simulink library "coeffs"  (R2014a)
settings: Solver=ode45  StartTime=0.0  StopTime=10.0  RelTol=1e-3
undefined symbols (not defined in the file or in its folder): par
settings Model: Creator=goghino  LastModifiedBy=goghino

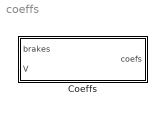
== system coeffs ==
  Coeffs : Subsystem

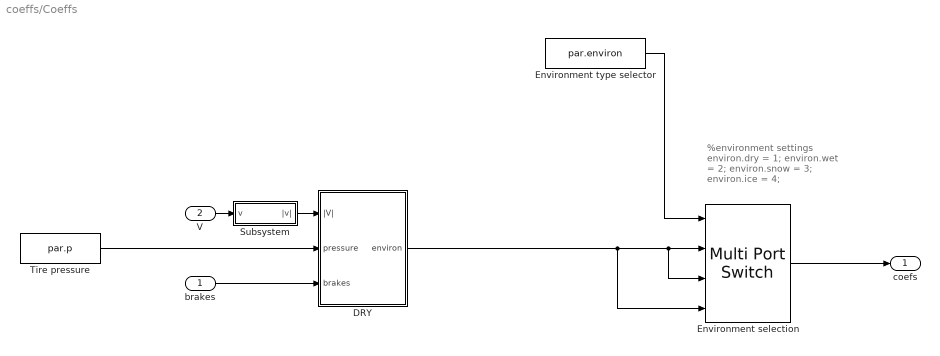
== system coeffs/Coeffs ==
  note: %environment settings
      | environ.dry = 1;
      | environ.wet = 2;
      | environ.snow = 3;
      | environ.ice = 4;
  brakes : Inport
  V : Inport  Port=2
  DRY : Subsystem
  Environment selection : MultiPortSwitch
  Environment type selector : Constant  Value=par.environ
  Subsystem : Subsystem
  Tire pressure : Constant  Value=par.p
  coefs : Outport
  wires:
  Environment selection/1 -> coefs/1
  Environment type selector/1 -> Environment selection/1
  DRY/1(environ) -> Environment selection/4, Environment selection/3, Environment selection/2
  V/1 -> Subsystem/1(v)
  Tire pressure/1 -> DRY/2(pressure)
  brakes/1 -> DRY/3(brakes)
  Subsystem/1(|v|) -> DRY/1(|V|)

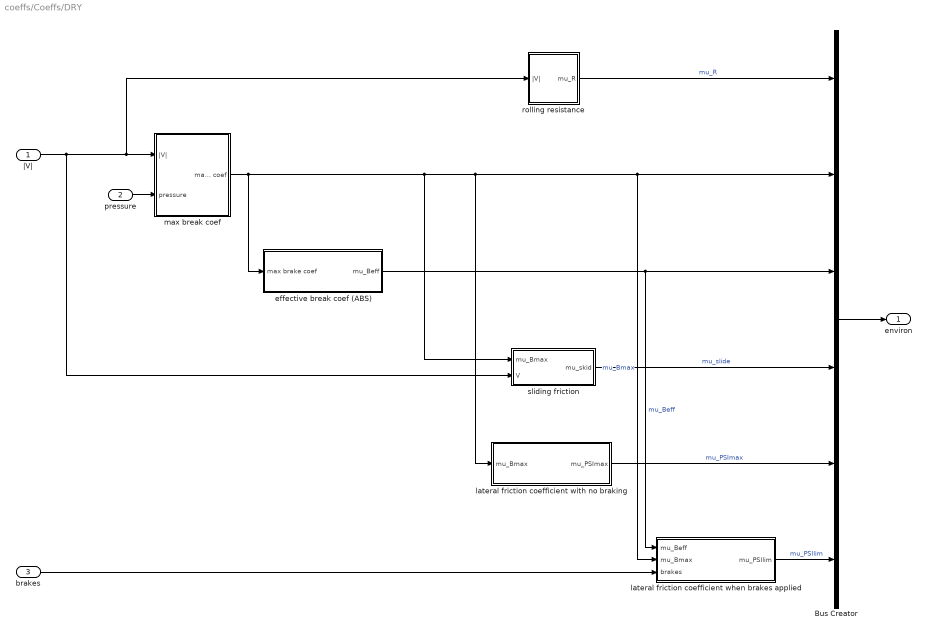
== system coeffs/Coeffs/DRY ==
  |V| : Inport
  pressure : Inport  Port=2
  brakes : Inport  Port=3
  Bus Creator : BusCreator  Inputs=6
  effective break coef (ABS) : Subsystem
  lateral friction coefficient when brakes applied : Subsystem
  lateral friction coefficient with no braking : Subsystem
  max break coef : Subsystem
  rolling resistance : Subsystem
  sliding friction : Subsystem
  environ : Outport
  wires:
  Bus Creator/1 -> environ/1
  pressure/1 -> max break coef/2(pressure)
  max break coef/1(max break coef) -> sliding friction/1(mu_Bmax), Bus Creator/2, lateral friction coefficient when brakes applied/2(mu_Bmax), lateral friction coefficient with no braking/1(mu_Bmax), effective break coef (ABS)/1(max brake coef)  "mu_Bmax"
  effective break coef (ABS)/1(mu_Beff) -> lateral friction coefficient when brakes applied/1(mu_Beff), Bus Creator/3  "mu_Beff"
  lateral friction coefficient with no braking/1(mu_PSImax) -> Bus Creator/5  "mu_PSImax"
  lateral friction coefficient when brakes applied/1(mu_PSIlim) -> Bus Creator/6  "mu_PSIlim"
  brakes/1 -> lateral friction coefficient when brakes applied/3(brakes)
  rolling resistance/1(mu_R) -> Bus Creator/1  "mu_R"
  |V|/1 -> sliding friction/2(V), rolling resistance/1(|V|), max break coef/1(|V|)
  sliding friction/1(mu_skid) -> Bus Creator/4  "mu_slide"

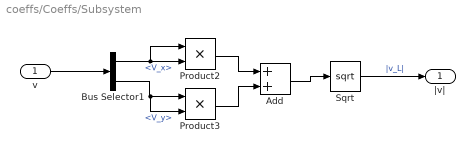
== system coeffs/Coeffs/Subsystem ==
  v : Inport
  Add : Sum
  Bus Selector1 : BusSelector  OutputSignals=V_x,V_y
  Product2 : Product
  Product3 : Product
  Sqrt : Sqrt  SaturateOnIntegerOverflow=on
  |v| : Outport
  wires:
  Add/1 -> Sqrt/1
  Product3/1 -> Add/2
  Bus Selector1/2 -> Product3/2, Product3/1  "<V_y>"
  v/1 -> Bus Selector1/1
  Bus Selector1/1 -> Product2/1, Product2/2  "<V_x>"
  Sqrt/1 -> |v|/1  "|v_L|"
  Product2/1 -> Add/1

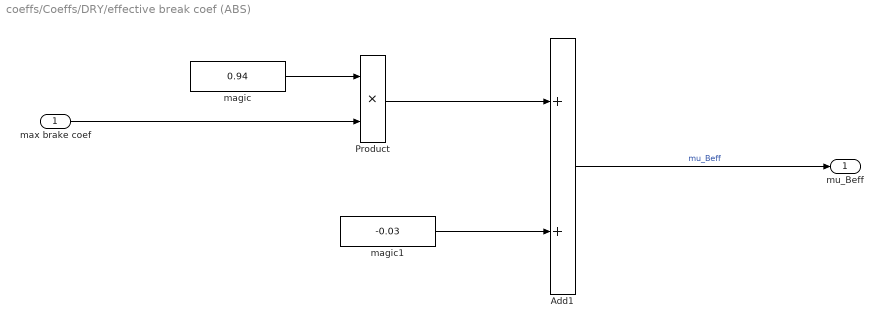
== system coeffs/Coeffs/DRY/effective break coef (ABS) ==
  max brake coef : Inport
  Add1 : Sum
  Product : Product
  magic : Constant  Value=0.94
  magic1 : Constant  Value=-0.03
  mu_Beff : Outport
  wires:
  Add1/1 -> mu_Beff/1  "mu_Beff"
  magic1/1 -> Add1/2
  max brake coef/1 -> Product/2
  magic/1 -> Product/1
  Product/1 -> Add1/1

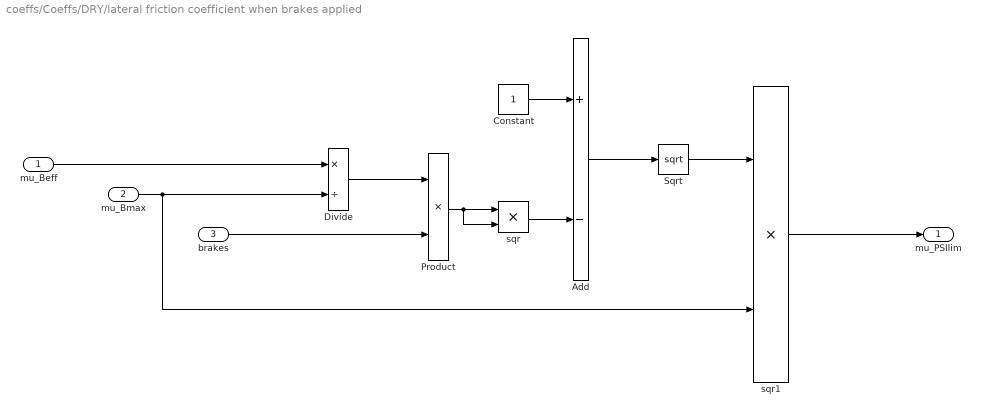
== system coeffs/Coeffs/DRY/lateral friction coefficient when brakes applied ==
  mu_Beff : Inport
  mu_Bmax : Inport  Port=2
  brakes : Inport  Port=3
  Add : Sum  Inputs=+-
  Constant : Constant
  Divide : Product  Inputs=*/
  Product : Product
  Sqrt : Sqrt  SaturateOnIntegerOverflow=on
  sqr : Product
  sqr1 : Product
  mu_PSIlim : Outport
  wires:
  Constant/1 -> Add/1
  Add/1 -> Sqrt/1
  mu_Beff/1 -> Divide/1
  mu_Bmax/1 -> sqr1/2, Divide/2
  Divide/1 -> Product/1
  brakes/1 -> Product/2
  sqr/1 -> Add/2
  Product/1 -> sqr/2, sqr/1
  Sqrt/1 -> sqr1/1
  sqr1/1 -> mu_PSIlim/1

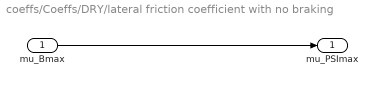
== system coeffs/Coeffs/DRY/lateral friction coefficient with no braking ==
  mu_Bmax : Inport
  mu_PSImax : Outport
  wires:
  mu_Bmax/1 -> mu_PSImax/1

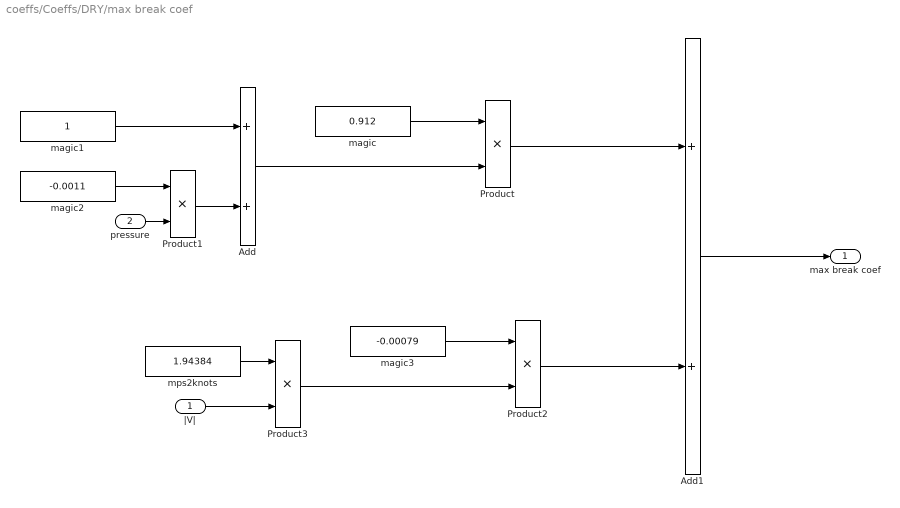
== system coeffs/Coeffs/DRY/max break coef ==
  |V| : Inport
  pressure : Inport  Port=2
  Add : Sum
  Add1 : Sum
  Product{,1..3} (4 alike) : Product
  magic : Constant  Value=0.912
  magic1 : Constant
  magic2 : Constant  Value=-0.0011
  magic3 : Constant  Value=-0.00079
  mps2knots : Constant  Value=1.94384
  max break coef : Outport
  wires:
  magic/1 -> Product/1
  magic1/1 -> Add/1
  Product1/1 -> Add/2
  magic2/1 -> Product1/1
  pressure/1 -> Product1/2
  Add/1 -> Product/2
  Product/1 -> Add1/1
  Product2/1 -> Add1/2
  magic3/1 -> Product2/1
  Add1/1 -> max break coef/1
  Product3/1 -> Product2/2
  mps2knots/1 -> Product3/1
  |V|/1 -> Product3/2

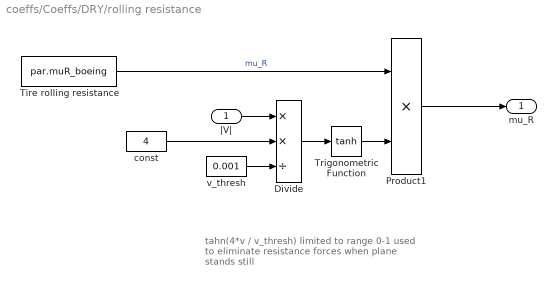
== system coeffs/Coeffs/DRY/rolling resistance ==
  note: tahn(4*v / v_thresh) limited to range 0-1
      | used to eliminate resistance forces
      | when plane stands still
  |V| : Inport
  Divide : Product  Inputs=**/
  Product1 : Product
  Tire rolling resistance : Constant  Value=par.muR_boeing
  Trigonometric Function : Trigonometry  Operator=tanh
  const : Constant  Value=4
  v_thresh : Constant  Value=0.001
  mu_R : Outport
  wires:
  Tire rolling resistance/1 -> Product1/1  "mu_R"
  v_thresh/1 -> Divide/3
  Divide/1 -> Trigonometric Function/1
  Trigonometric Function/1 -> Product1/2
  Product1/1 -> mu_R/1
  |V|/1 -> Divide/1
  const/1 -> Divide/2

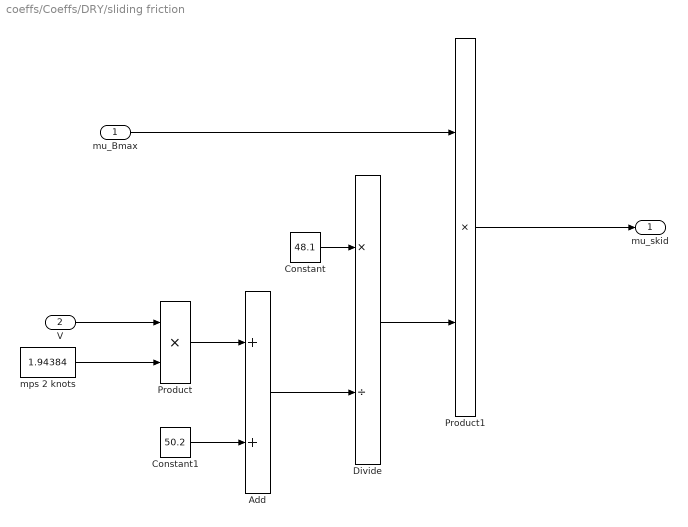
== system coeffs/Coeffs/DRY/sliding friction ==
  mu_Bmax : Inport
  V : Inport  Port=2
  Add : Sum
  Constant : Constant  Value=48.1
  Constant1 : Constant  Value=50.2
  Divide : Product  Inputs=*/  SaturateOnIntegerOverflow=on  RndMeth=Zero
  Product : Product
  Product1 : Product
  mps 2 knots : Constant  Value=1.94384
  mu_skid : Outport
  wires:
  Constant/1 -> Divide/1
  Product/1 -> Add/1
  Constant1/1 -> Add/2
  V/1 -> Product/1
  mps 2 knots/1 -> Product/2
  Add/1 -> Divide/2
  Divide/1 -> Product1/2
  mu_Bmax/1 -> Product1/1
  Product1/1 -> mu_skid/1
